simulink model "SERBERMPAM"  (R2017a)
settings: Solver=VariableStepDiscrete  StartTime=0.0  StopTime=time  RelTol=1e-3
values from neighbouring files (symbols this model uses):
  hrn = ones(1,OSF)/OSF    [scriptMPAMBB.m]
undefined symbols (not defined in the file or in its folder): fdesignblkfcn, gcbh
libraries: commdigbbndam3 x2, commchan3 x1, commrandsrc3 x1, commsink2 x1, commfilt2 x1
settings Model: Creator=Fabio  LastModifiedBy=Fabio
settings DataIOCC: LimitDataPoints=on  SaveOutput=off  SaveTime=off
settings OptimizationCC: BooleanDataType=off  DefaultParameterBehavior=Inlined  LocalBlockOutputs=off  LifeSpan=inf
settings DebuggingCC: AlgebraicLoopMsg=error  SingleTaskRateTransMsg=error  AllowSymbolicDim=off  SFUnexpectedBacktrackingDiag=warning  SFNoUnconditionalDefaultTransitionDiag=warning  SFExecutionAtInitializationDiag=none
settings GRTTargetCC: TargetLangStandard=C89/C90 (ANSI)  GeneratePreprocessorConditionals=Disable all
settings ConfigComp: CovMetricSettings=dw  CovHtmlReporting=on  CovSaveCumulativeToWorkspaceVar=on  CovSaveSingleToWorkspaceVar=on  CovExternalEMLEnable=off  CovSFcnEnable=off

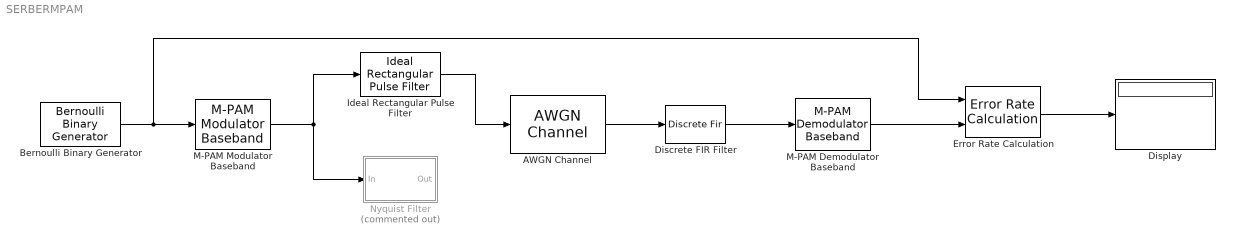
== system SERBERMPAM ==
  AWGN Channel : commchan3/AWGN Channel  InputProcessing=Columns as channels (frame based)  seed=67  noiseMode="Signal to noise ratio  (Eb/No)"  EbNodB=10  EsNodB=10  SNRdB=10  bitsPerSym=1  Ps=1  Tsym=1  variance=1
  Bernoulli Binary Generator : commrandsrc3/Bernoulli Binary Generator  ProbabilityOfZero=0.5  SeedSource=Auto  Seed=0  SampleTime=1  SamplesPerFrame=1  OutputDataType=double  SimulateUsing=Interpreted execution
  Discrete FIR Filter : DiscreteFir  Coefficients=hrn
  Display : Display
  Error Rate Calculation : commsink2/Error Rate Calculation  N=0  st_delay=0  cp_mode=Entire frame  subframe=[]  PMode=Port  WsName=ErrorVec  RsMode2=off  stop=off  numErr=100  maxBits=1e6
  Ideal Rectangular Pulse Filter : commfilt2/Ideal Rectangular Pulse Filter  pulseLen=8  pulseDelay=0  InputProcessing=Columns as channels (frame based)  RateOptions=Enforce single-rate processing  sampMode=Mute  normCheck=off  normMode=Sum of samples  filterGain=1  saveAsFlag=0  roundingMode=Floor  overflowMode=off  firstCoeffDataTypeStr=Inherit: Same word length as input  firstCoeffMin=[]  firstCoeffMax=[]  firstCoeffLastDataTypeStr=Inherit: Same word length as input  outputDataTypeStr=Inherit: Same as accumulator  outputMin=[]  outputMax=[]  outputLastDataTypeStr=Inherit: Same as accumulator
      settings: SourceProductName=Communications System Toolbox  SourceProductBaseCode=CM
  M-PAM Demodulator Baseband : commdigbbndam3/M-PAM Demodulator Baseband  M=4  OutType=Integer  Dec=Gray  PowType=Min. distance between symbols  MinDist=2  AvgPow=1  PeakPow=1  outDtype1=Inherit via internal rule  outDtype2=Inherit via internal rule  denormFactorWordLen=16  denormFactorDataTypeStr=Inherit: Same word length as input  denormFactorLastDataTypeStr=Inherit: Same word length as input  prodOutWordLen=16  prodOutRoundingMode=Floor  prodOutOverflowMode=Wrap  prodOutOvFlMode=off  prodOutOvFlModeLastStrValue=off  sumWordLen=16
      settings: SourceProductName=Communications System Toolbox  SourceProductBaseCode=CM
  M-PAM Modulator Baseband : commdigbbndam3/M-PAM Modulator Baseband  M=4  InType=Integer  Enc=Gray  PowType=Min. distance between symbols  MinDist=2  AvgPow=1  PeakPow=1  outDtype=double  outWordLen=16  outUDDataType=sfix(16)  outFracLenMode=Best precision  outFracLen=15  outDataTypeStr=double  outLastDataTypeStr=double
      settings: SourceProductName=Communications System Toolbox  SourceProductBaseCode=CM
  Nyquist Filter : Subsystem  Commented=on  DialogController=fdesignblkfcn  InitFcn=fdesignblkfcn(gcbh, {'InitFcn'});  mask(Nyquist Filter){}
      mask help: Design a Nyquist filter
      settings: CopyFcn=fdesignblkfcn(gcbh, {'CopyFcn'});
      mask Help: helpview(mapfilelocation('dsp'), 'dspnyquistfilter');
      mask Display: disp('Nyquist');
  wires:
  Bernoulli Binary Generator/1 -> Error Rate Calculation/1, M-PAM Modulator Baseband/1
  M-PAM Modulator Baseband/1 -> Nyquist Filter/1(In), Ideal Rectangular Pulse Filter/1
  Ideal Rectangular Pulse Filter/1 -> AWGN Channel/1
  AWGN Channel/1 -> Discrete FIR Filter/1
  Discrete FIR Filter/1 -> M-PAM Demodulator Baseband/1
  M-PAM Demodulator Baseband/1 -> Error Rate Calculation/2
  Error Rate Calculation/1 -> Display/1

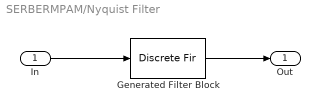
== system SERBERMPAM/Nyquist Filter ==
  In : Inport
  Generated Filter Block : DiscreteFir  Tag=BlockMethodSubSystem  Coefficients=[-1.5162272612995586e-05 0 4.1706564279713027e-05 0 -8.6397453235949307e-05 0 0.00015611233941239259 0 -0.00025915216340561289 0 0.00040534096772710702 0 -0.00060612208112690072 0 0.00087466461351889491 0 -0.0012260032157642615 0 0.0016772472887656247 0 -0.0022479153417375975 0 0.002960480176087802 0 -0.0038412587047380814 0 0.0049218611113159959 0 -0.0062415564318662039 0 0.0078511744671022864 0 -0.0098196745838436145 0 0.012245562776669343 0 -0.015277650505299337 0 0.019155163922055268 0 -0.024291754943524414 0 0.031471599148898237 0 -0.042381607242685339 0 0.061420660829271646 0 -0.10474499179295332 0 0.31785484611193615 0.5 0.31785484611193615 0 -0.10474499179295332 0 0.061420660829271646 0 -0.042381607242685339 0 0.031471599148898237 0 -0.024291754943524414 0 0.019155163922055268 0 -0.015277650505299337 0 0.012245562776669343 0 -0.0098196745838436145 0 0.0078511744671022864 0 -0.0062415564318662039 0 0.0049218611113159959 0 -0.0038412587047380814 0 0.002960480176087802 0 -0.0022479153417375975 0 0.0016772472887656247 0 -0.0012260032157642615 0 0.00087466461351889491 0 -0.00060612208112690072 0 0.00040534096772710702 0 -0.00025915216340561289 0 0.00015611233941239259 0 -8.6397453235949307e-05 0 4.1706564279713027e-05 0 -1.5162272612995586e-05]  InputProcessing=Columns as channels (frame based)
  Out : Outport
  wires:
  In/1 -> Generated Filter Block/1
  Generated Filter Block/1 -> Out/1
